simulink model "case_36_mode0_lead_oscillates_12"  (R2025b)
settings: Solver=VariableStepAuto  StartTime=0.0  StopTime=15  RelTol=1e-3
model workspace (MAT data in the model file):
  Amplitude = 1
settings Model: Creator=sanborkl  LastModifiedBy=admin

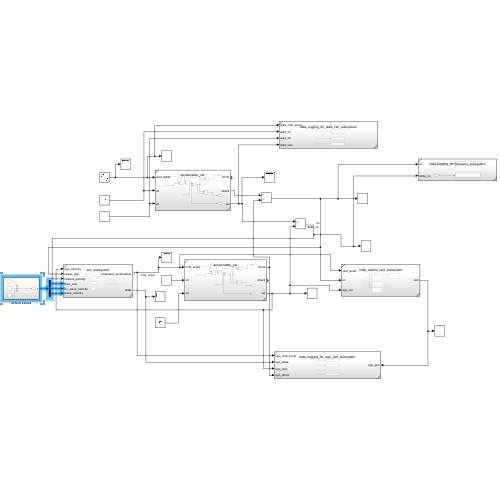
[thumbnail: Simulink's stored preview of the top-level diagram]
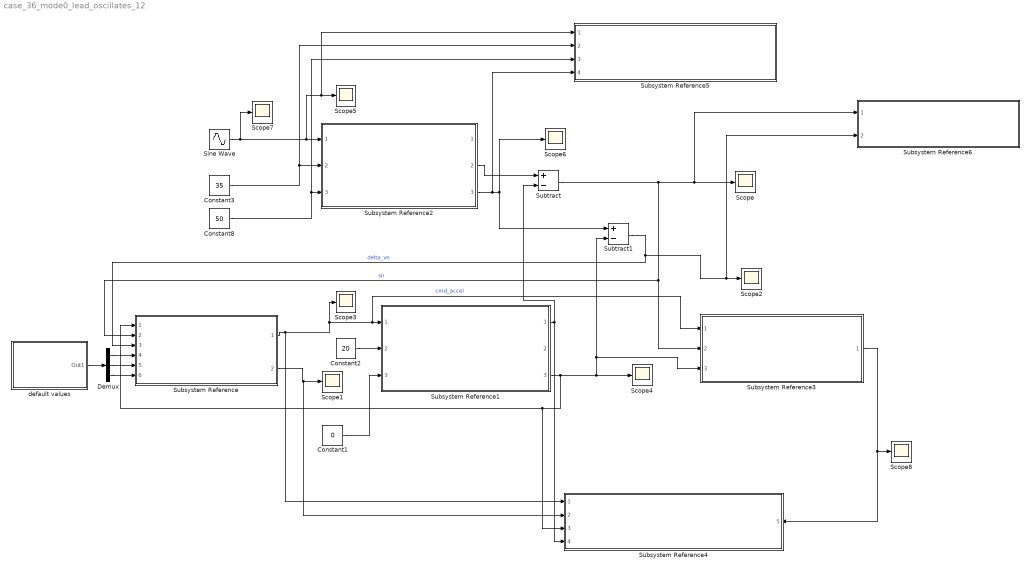
== system case_36_mode0_lead_oscillates_12 ==
  Constant1 : Constant  Value=0
  Constant2 : Constant  Value=20
  Constant3 : Constant  Value=35
  Constant8 : Constant  Value=50
  Demux : Demux  Outputs=3
  Scope{,1..8} (9 alike) : Scope
      Scope settings: ActiveDisplayYMinimum=-1  ActiveDisplayYMaximum=1
      Scope1 settings: ActiveDisplayYMinimum=-1  ActiveDisplayYMaximum=1  DataLoggingVariableName=ScopeData2
      Scope2 settings: ActiveDisplayYMinimum=-2.4298440672339487  ActiveDisplayYMaximum=0.26998267413710536  DataLoggingVariableName=ScopeData3
      Scope3 settings: ActiveDisplayYMinimum=-0.18749999999999994  ActiveDisplayYMaximum=1.6875  DataLoggingVariableName=ScopeData4
      Scope4 settings: ActiveDisplayYMinimum=-1  ActiveDisplayYMaximum=1
      Scope5 settings: ActiveDisplayYMinimum=-1.7936866858199967  ActiveDisplayYMaximum=1.7717792887568067  DataLoggingVariableName=ScopeData5
      Scope6 settings: ActiveDisplayYMinimum=19.945608533557348  ActiveDisplayYMaximum=20.489523197983868  DataLoggingVariableName=ScopeData6
      Scope7 settings: ActiveDisplayYMinimum=-0.24995828372720832  ActiveDisplayYMaximum=0.24962499487656459  DataLoggingVariableName=ScopeData7
      Scope8 settings: ActiveDisplayYMinimum=-0.12499999999999997  ActiveDisplayYMaximum=1.125  DataLoggingVariableName=ScopeData8
  Sine Wave : Sin  Frequency=2 * pi * 1  SampleTime=0
  Subsystem Reference : Subsystem  ReferencedSubsystem=acc_subsystem
  Subsystem Reference1 : Subsystem  ReferencedSubsystem=acceleration_car
  Subsystem Reference2 : Subsystem  ReferencedSubsystem=acceleration_car
  Subsystem Reference3 : Subsystem  ReferencedSubsystem=multi_vehicle_test_subsystem
  Subsystem Reference4 : Subsystem  ReferencedSubsystem=data_logging_for_ego_veh_subsystem
      settings: PortSchema="{\"entries\":[{\"content\":{\"sides\":[{\"content\":{\"connectorIds\":[\"In1\",\"In2\",\"In3\",\"In4\"]},\"type\":\"ConnectorPlacement.EquallySpacedRectSide\",\"uuid\":\"1bb3a8cf-f981-4f8a-aff9-03896ccf7d7c\"},{\"content\":{\"connectorIds\":[\"In5\"],\"side\":\"RIGHT\"},\"type\":\"ConnectorPlacement.EquallySpacedRectSide\",\"uuid\":\"3f6ac5cb-96be-44a3-8993-3635a91bd658\"},{\"content\":{\"side\":\"TOP\"},\"type\":\"ConnectorPlacement.EquallySpacedRectSide\",\"uuid\":\"c641fc7f-a424-4033-b273-2526f6b205c0\"}]},\"type\":\"ConnectorPlacement.EquallySpacedConnector\",\"uuid\":\"2a4be48e-084e-4aa6-b74f-8fe234fedc1a\"}],\"packageUris\":[\"http://schema.mathworks.com/mf0/Connector/R2020b\"],\"version\":\"1.0\"}"
  Subsystem Reference5 : Subsystem  ReferencedSubsystem=data_logging_for_lead_veh_subsystem
  Subsystem Reference6 : Subsystem  ReferencedSubsystem=data_logging_for_behavior_subsystem
  Subtract : Sum  Inputs=+-
  Subtract1 : Sum  Inputs=+-
  default values : Subsystem
  wires:
  Subsystem Reference2/3 -> Subsystem Reference5/4, Scope6/1, Subtract1/1
  Constant3/1 -> Subsystem Reference5/2, Subsystem Reference2/2
  Constant2/1 -> Subsystem Reference1/2
  Subsystem Reference/1 -> Subsystem Reference4/1, Scope3/1, Subsystem Reference3/1, Subsystem Reference1/1  "cmd_accel"
  Constant1/1 -> Subsystem Reference1/3
  Subsystem Reference/2 -> Subsystem Reference4/2, Scope1/1
  Subsystem Reference2/2 -> Subtract/1
  Subtract/1 -> Subsystem Reference3/2, Subsystem Reference/2, Subsystem Reference6/1, Scope/1  "sn"
  Subsystem Reference1/3 -> Subsystem Reference4/3, Subsystem Reference/1, Subtract1/2, Subsystem Reference3/3, Scope4/1
  Subtract1/1 -> Subsystem Reference6/2, Scope2/1, Subsystem Reference/3  "delta_vn"
  Constant8/1 -> Subsystem Reference5/3, Subsystem Reference2/3
  Sine Wave/1 -> Scope7/1, Subsystem Reference5/1, Scope5/1, Subsystem Reference2/1
  Subsystem Reference1/1 -> Subtract/2, Subsystem Reference4/4
  Subsystem Reference3/1 -> Scope8/1, Subsystem Reference4/5
  Demux/3 -> Subsystem Reference/6
  Demux/2 -> Subsystem Reference/5
  default values/1(Out1) -> Demux/1
  Demux/1 -> Subsystem Reference/4

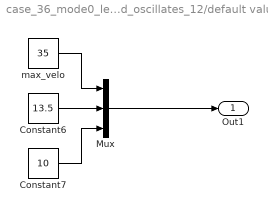
== system case_36_mode0_lead_oscillates_12/default values ==
  Constant6 : Constant  Value=13.5
  Constant7 : Constant  Value=10
  Mux : Mux  Inputs=3
  max_velo : Constant  Value=35
  Out1 : Outport
  wires:
  Constant7/1 -> Mux/3
  Constant6/1 -> Mux/2
  max_velo/1 -> Mux/1
  Mux/1 -> Out1/1
